simulink model "COMPTORQUE_Amato_spaziogiunti"  (R2018b)
settings: Solver=FixedStepAuto  StartTime=0.0  StopTime=50  FixedStep=t_c  RelTol=1e-3
values from neighbouring files (symbols this model uses):
  A_circolare_com = 0.1    [Init.m]    (also in WS_regressor.mat)
  A_circolare_hand = 0.005    [Init.m]    (also in WS_regressor.mat = 0.0005)
  cond_init = [x1,x2,x3,x4,x5,x6]'    [Init.m]    (also in WS_regressor.mat = [0.523598775598 2.09439510239 -1.0471975512 1.57079632679 1.)
  Law = [kp, kd]    [Init.m]    (also in LAUNCH_Backstepping.m = [lambda, kd]; LAUNCH_Backstepping_adapt.m = [K_lambda, K_d, K_r]; LAUNCH_CToque.m; WS_regressor.mat = [500 50])
  param = param'    [Init.m]    (also in WS_regressor.mat = [1 1 1 1 1 1 0 1 1 1 3 3 ... (14 elements, 7x2)])
  pulsazione_circolare = 1    [Init.m]    (also in WS_regressor.mat)
  x0 = -1.5    [Init.m]    (also in WS_regressor.mat)
  y0 = 2    [Init.m]    (also in WS_regressor.mat)
libraries: simulink x2
settings Model: Creator=AmatoPi  LastModifiedBy=Utente

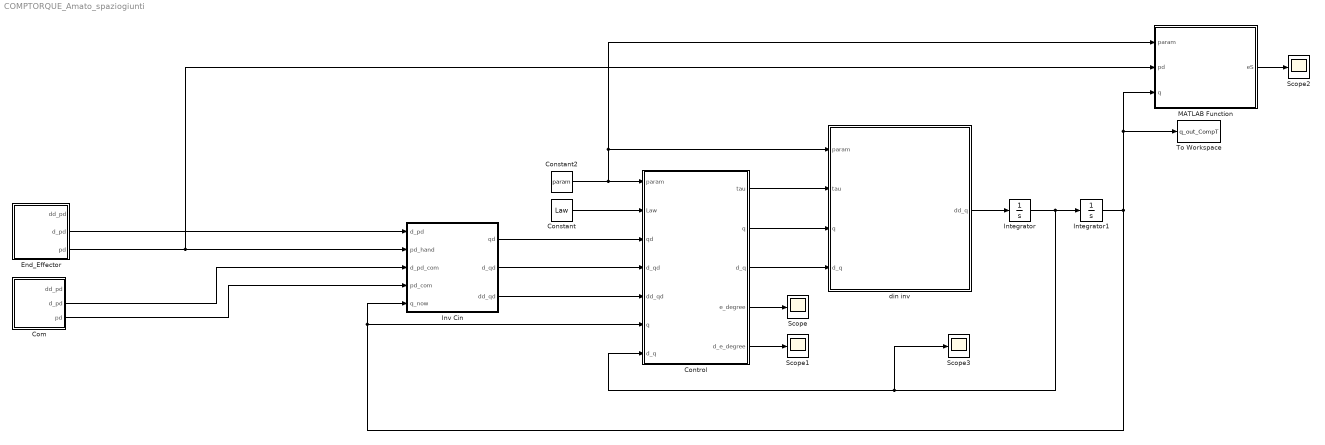
== system COMPTORQUE_Amato_spaziogiunti ==
  Com : Subsystem
  Constant : Constant  Value=Law
  Constant2 : Constant  Value=param
  Control : MATLAB Function  TreatAsAtomicUnit=on
  End_Effector : Subsystem
  Integrator : Integrator  InitialCondition=[0,0,0,0,0,0]'
  Integrator1 : Integrator  InitialCondition=cond_init
  Inv Cin : Subsystem
  MATLAB Function : MATLAB Function  TreatAsAtomicUnit=on
  Scope{,1..3} (4 alike) : Scope
  To Workspace : ToWorkspace  VariableName=q_out_CompT  SaveFormat=Structure With Time  SampleTime=-1
  din inv : MATLAB Function  TreatAsAtomicUnit=on
  wires:
  End_Effector/2(d_pd) -> Inv Cin/1(d_pd)
  End_Effector/3(pd) -> MATLAB Function/2(pd), Inv Cin/2(pd_hand)
  Inv Cin/1(qd) -> Control/3(qd)
  Inv Cin/2("d_qd ") -> Control/4(d_qd)
  Inv Cin/3(dd_qd) -> Control/5(dd_qd)
  Constant/1 -> Control/2(Law)
  Constant2/1 -> MATLAB Function/1(param), din inv/1(param), Control/1(param)
  Control/1(tau) -> din inv/2(tau)
  Control/2(q) -> din inv/3(q)
  Control/3(d_q) -> din inv/4(d_q)
  din inv/1(dd_q) -> Integrator/1
  Integrator/1 -> Control/7("d_q "), Scope3/1, Integrator1/1
  Integrator1/1 -> Inv Cin/5(q_now), Control/6("q "), MATLAB Function/3(q), To Workspace/1
  Control/4(e_degree) -> Scope/1
  Control/5(d_e_degree) -> Scope1/1
  MATLAB Function/1(eS) -> Scope2/1
  Com/2(d_pd) -> Inv Cin/3(d_pd_com)
  Com/3(pd) -> Inv Cin/4(pd_com)

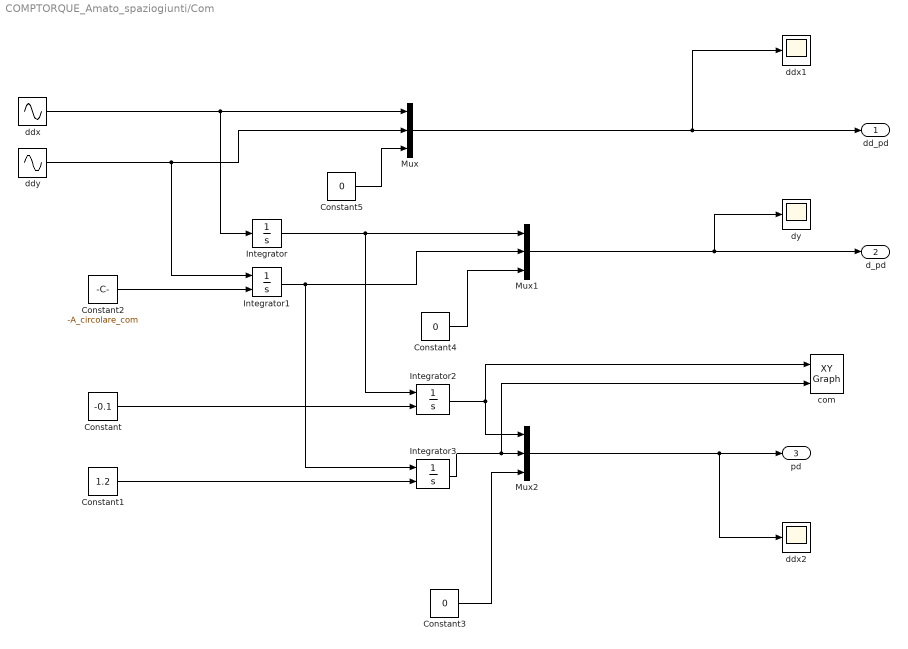
== system COMPTORQUE_Amato_spaziogiunti/Com ==
  Constant : Constant  Value=-0.1
  Constant1 : Constant  Value=1.2
  Constant2 : Constant  Value=-A_circolare_com
  Constant3 : Constant  Value=0
  Constant4 : Constant  Value=0
  Constant5 : Constant  Value=0
  Integrator : Integrator
  Integrator1 : Integrator  InitialConditionSource=external
  Integrator2 : Integrator  InitialConditionSource=external
  Integrator3 : Integrator  InitialConditionSource=external
  Mux : Mux  Inputs=3
  Mux1 : Mux  Inputs=3
  Mux2 : Mux  Inputs=3
  com : simulink/Sinks/XY Graph  xmin=xL  xmax=xR  ymin=yD  ymax=yU  st=-1
  ddx : Sin  Amplitude=A_circolare_com  Frequency=pulsazione_circolare  Phase=pi/2  SampleTime=0
  ddx1 : Scope
  ddx2 : Scope
  ddy : Sin  Amplitude=A_circolare_com  Frequency=pulsazione_circolare  SampleTime=0
  dy : Scope
  dd_pd : Outport
  d_pd : Outport  Port=2
  pd : Outport  Port=3
  wires:
  ddx/1 -> Integrator/1, Mux/1
  ddy/1 -> Mux/2, Integrator1/1
  Integrator2/1 -> com/1, Mux2/1
  Integrator/1 -> Integrator2/1, Mux1/1
  Integrator3/1 -> com/2, Mux2/2
  Integrator1/1 -> Integrator3/1, Mux1/2
  Constant/1 -> Integrator2/2
  Constant1/1 -> Integrator3/2
  Constant2/1 -> Integrator1/2
  Constant3/1 -> Mux2/3
  Constant4/1 -> Mux1/3
  Constant5/1 -> Mux/3
  Mux/1 -> ddx1/1, dd_pd/1
  Mux1/1 -> dy/1, d_pd/1
  Mux2/1 -> ddx2/1, pd/1

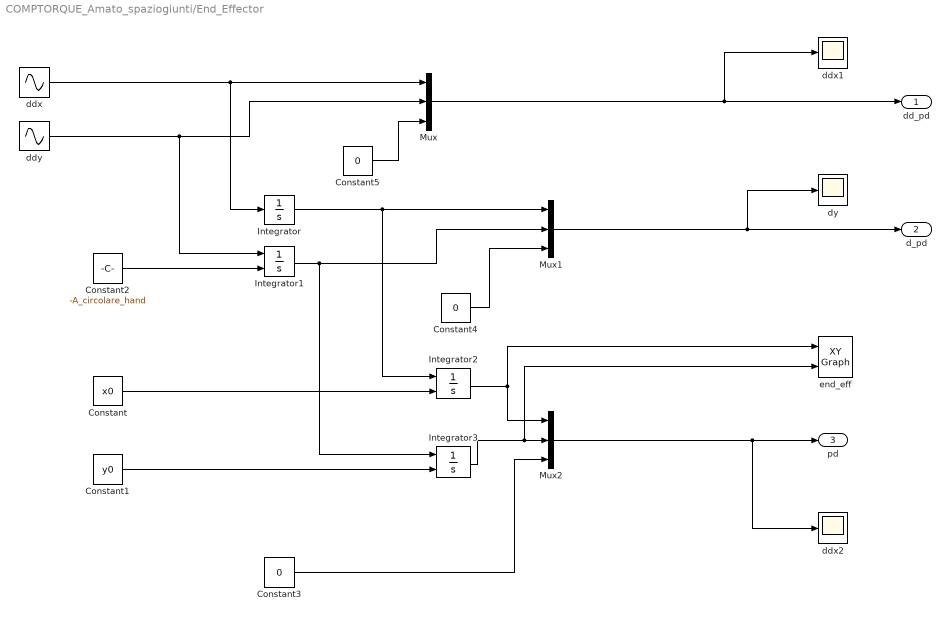
== system COMPTORQUE_Amato_spaziogiunti/End_Effector ==
  Constant : Constant  Value=x0
  Constant1 : Constant  Value=y0
  Constant2 : Constant  Value=-A_circolare_hand
  Constant3 : Constant  Value=0
  Constant4 : Constant  Value=0
  Constant5 : Constant  Value=0
  Integrator : Integrator
  Integrator1 : Integrator  InitialConditionSource=external
  Integrator2 : Integrator  InitialConditionSource=external
  Integrator3 : Integrator  InitialConditionSource=external
  Mux : Mux  Inputs=3
  Mux1 : Mux  Inputs=3
  Mux2 : Mux  Inputs=3
  ddx : Sin  Amplitude=-A_circolare_hand  Frequency=pulsazione_circolare  Phase=pi/2  SampleTime=0
  ddx1 : Scope
  ddx2 : Scope
  ddy : Sin  Amplitude=A_circolare_hand  Frequency=pulsazione_circolare  SampleTime=0
  dy : Scope
  end_eff : simulink/Sinks/XY Graph  xmin=xL  xmax=xR  ymin=yD  ymax=yU  st=-1
  dd_pd : Outport
  d_pd : Outport  Port=2
  pd : Outport  Port=3
  wires:
  ddx/1 -> Integrator/1, Mux/1
  ddy/1 -> Mux/2, Integrator1/1
  Integrator2/1 -> end_eff/1, Mux2/1
  Integrator/1 -> Integrator2/1, Mux1/1
  Integrator3/1 -> end_eff/2, Mux2/2
  Integrator1/1 -> Integrator3/1, Mux1/2
  Constant/1 -> Integrator2/2
  Constant1/1 -> Integrator3/2
  Constant2/1 -> Integrator1/2
  Constant3/1 -> Mux2/3
  Constant4/1 -> Mux1/3
  Constant5/1 -> Mux/3
  Mux/1 -> ddx1/1, dd_pd/1
  Mux1/1 -> dy/1, d_pd/1
  Mux2/1 -> ddx2/1, pd/1

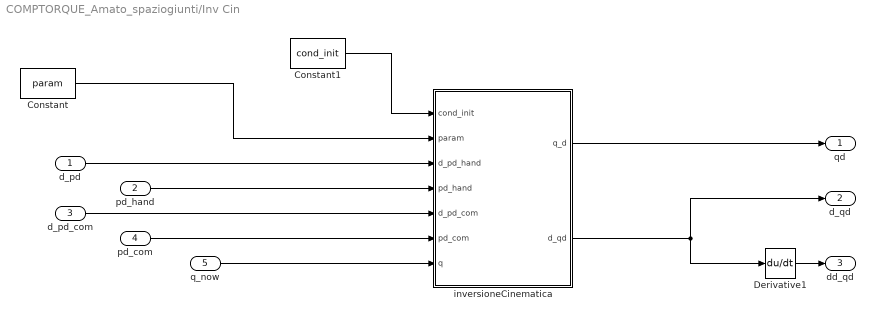
== system COMPTORQUE_Amato_spaziogiunti/Inv Cin ==
  d_pd : Inport
  pd_hand : Inport  Port=2
  d_pd_com : Inport  Port=3
  pd_com : Inport  Port=4
  q_now : Inport  Port=5
  Constant : Constant  Value=param
  Constant1 : Constant  Value=cond_init
  Derivative1 : Derivative
  inversioneCinematica : MATLAB Function  TreatAsAtomicUnit=on
  qd : Outport
  "d_qd " : Outport  Port=2
  dd_qd : Outport  Port=3
  wires:
  Constant1/1 -> inversioneCinematica/1(cond_init)
  pd_hand/1 -> inversioneCinematica/4(pd_hand)
  Constant/1 -> inversioneCinematica/2(param)
  d_pd/1 -> inversioneCinematica/3(d_pd_hand)
  Derivative1/1 -> dd_qd/1
  inversioneCinematica/2(d_qd) -> Derivative1/1, "d_qd "/1
  pd_com/1 -> inversioneCinematica/6(pd_com)
  d_pd_com/1 -> inversioneCinematica/5(d_pd_com)
  q_now/1 -> inversioneCinematica/7(q)
  inversioneCinematica/1(q_d) -> qd/1

== matlab function COMPTORQUE_Amato_spaziogiunti/Control ==
  data: param input; Law input; tau output; qd input; d_qd input; dd_qd input; q input; d_q input; q output; d_q output; e_degree output; d_e_degree output
function [tau,q,d_q,e_degree,d_e_degree] = controlLaw(param,Law,qd,d_qd,dd_qd, q, d_q)

    d_e = d_qd - d_q;
    e = qd - q;

    kv = Law(2)*eye(6);
    kp = Law(1)*eye(6);

    [B,C,G] = Dinamica(param,q,d_q);

    tau = B*(dd_qd + kv*d_e + kp*e) + C*d_q + G;
    e_degree = e*180/pi;
    d_e_degree = d_e*180/pi;
end

== matlab function COMPTORQUE_Amato_spaziogiunti/Inv Cin/inversioneCinematica ==
  data: q_d output; cond_init input; param input; d_pd_hand input; pd_hand input; d_pd_com input; pd_com input; d_qd output; q input
function [q_d, d_qd]  = inv_cinematica(cond_init, param, d_pd_hand, pd_hand, d_pd_com,pd_com, q)
    
    %per ottenere qd e dd_qd devo per forza ricorrere a derivazione ed
    %integrazione
    
    des_hand = pd_hand;
    d_des_hand = d_pd_hand;
    
    des_com = pd_com;
    d_des_com = d_pd_com;
    
    J_c = J_com_fun(q);
    J_ha = J_hand_fun(q);
    
%     [~,des_com,~] = Direct_Kinematics(param,cond_init);
    
    %priorità di compito
    [p,com,~] = Direct_Kinematics(param,q);
    
    hand = p(6,:)';
    
    pinv_J_ha = pinv(J_ha);
    pinv_J_c = pinv(J_c);
     
%     pinv_J_c = pinv(J_c);
%     projN_J_c = eye(6) - pinv_J_c*J_c;
%     
%     Kc = 0.5;
%     Kha = 0.5;    
%     dq_com = pinv_J_c * Kc * (des_com-com);
%     dq_hand = projN_J_c * pinv_J_ha * ( d_des_hand + Kha * (des_hand-hand));
%     d_qd = dq_com + dq_hand;
% 
    I = eye(6);
    erroc_com = des_com - com;
%     J2tilde_pinv = pinv(J_c*(I-pinv_J_ha*J_ha));
    J2tilde_pinv = pinv(J_ha*(I-pinv_J_c*J_c));
    
    %Priorità alla mano che deve rimanere ferma.
%     d_qd = 0.5*(pinv_J_ha*(pd_hand-hand) + 0.5*(I - pinv_J_ha*J_ha)*J2tilde_pinv*(dy-J_c*pinv_J_ha*(pd_hand-hand)));
    d_qd = (pinv_J_c*erroc_com) + (I - pinv_J_c*J_c)*J2tilde_pinv*((pd_hand-hand)-J_ha*pinv_J_c*erroc_com);
    q_d = q + 0.01*d_qd;
    
    
%     d_qd = pinv_J_c*dy;
%     q_d = q + 0.01*d_qd;


%     d_qd = pinv_J_ha*d_pd_hand + (I - pinv_J_ha*J_ha)*J2tilde_pinv*(d_des_com-J_c*pinv_J_ha*d_pd_hand);

%     q_d = q + 0.1*(J_c')*(pd-com);
%     q_d = q + 0.1*pinv_J_ha*(pd-hand);
%     d_qd = pinv_J_c*d_pd;

    
end

== matlab function COMPTORQUE_Amato_spaziogiunti/din inv ==
  data: param input; tau input; dd_q output; q input; d_q input
function dd_q = dinamica_inv(param,tau,q,d_q)

[B,C,G] = Dinamica(param,q,d_q);

dd_q = B\(tau - C*d_q - G);

end

== matlab function COMPTORQUE_Amato_spaziogiunti/MATLAB Function ==
  data: param input; pd input; q input; eS output
function eS = error_SpazioOperativo(param,pd,q)

    [p,com,~] = Direct_Kinematics(param,q);
    
    eS = pd-p(6,:)';

end
